simulink model "SimulationOfFurutaL"  (R2017a)
settings: Solver=ode5  StartTime=0.0  StopTime=20  FixedStep=0.0001  RelTol=1e-3  EnableMultiTasking=on
settings Model: Creator=marce  LastModifiedBy=felip
settings DataIOCC: LimitDataPoints=on  SaveFormat=Array
settings OptimizationCC: LifeSpan=inf
settings DebuggingCC: SFUnexpectedBacktrackingDiag=warning  SFNoUnconditionalDefaultTransitionDiag=warning  SFExecutionAtInitializationDiag=none
settings HardwareCC: ProdBitPerPointer=32  ProdBitPerSizeT=32  ProdBitPerPtrDiffT=32  ProdLargestAtomicFloat=None  ProdIntDivRoundTo=Undefined  ProdEndianess=Unspecified  ProdWordSize=32  ProdHWDeviceType=32-bit Generic
settings ModelReferenceCC: PropagateSignalLabelsOutOfModel=off
settings GRTTargetCC: TargetLangStandard=C89/C90 (ANSI)  GeneratePreprocessorConditionals=Disable all
settings ConfigComp: CovMetricSettings=dw  CovHtmlReporting=on  CovSaveCumulativeToWorkspaceVar=on  CovSaveSingleToWorkspaceVar=on  CovExternalEMLEnable=off

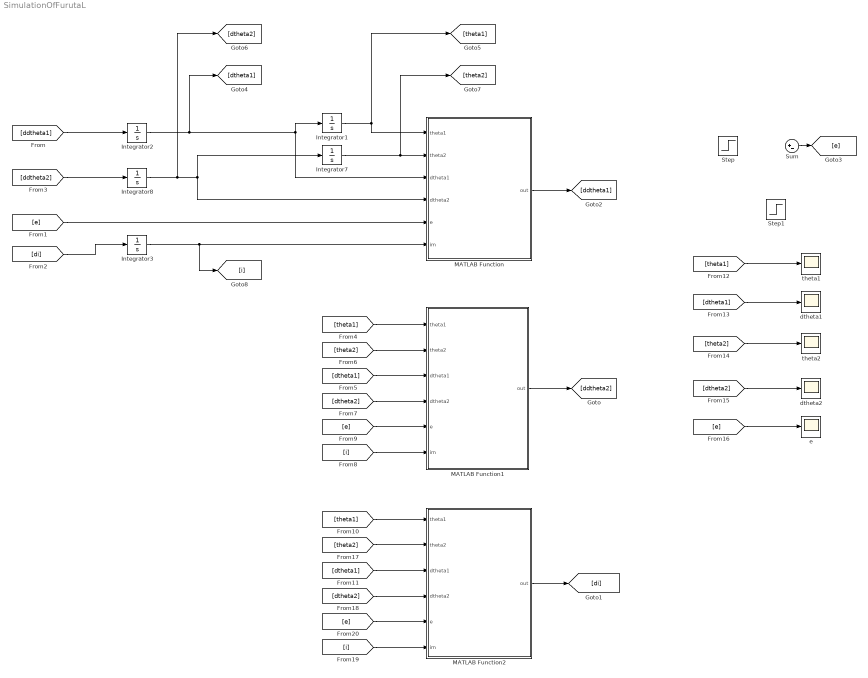
== system SimulationOfFurutaL ==
  Integrator{1..3,8} (4 alike) : Integrator
  Integrator7 : Integrator  InitialCondition=pi*15/180
  MATLAB Function : MATLAB Function  TreatAsAtomicUnit=on
  MATLAB Function1 : MATLAB Function  TreatAsAtomicUnit=on
  MATLAB Function2 : MATLAB Function  TreatAsAtomicUnit=on
  Step : Step  Time=0  After=12  SampleTime=0
  Step1 : Step  Time=1/12  After=12  SampleTime=0
  Sum : Sum  Inputs=|+-
  dtheta1 : Scope
  dtheta2 : Scope
  e : Scope
  theta1 : Scope
  theta2 : Scope
  wires:
  MATLAB Function/1(out) -> [ddtheta1]
  MATLAB Function2/1(out) -> [di]
  MATLAB Function1/1(out) -> [ddtheta2]
  [ddtheta1] -> Integrator2/1
  [ddtheta2] -> Integrator8/1
  Integrator8/1 -> Integrator7/1, MATLAB Function/4(dtheta2), [dtheta2]
  Integrator7/1 -> [theta2], MATLAB Function/2(theta2)
  Sum/1 -> [e]
  Integrator1/1 -> MATLAB Function/1(theta1), [theta1]
  [theta1] -> theta1/1
  [dtheta1] -> dtheta1/1
  [theta2] -> theta2/1
  [dtheta2] -> dtheta2/1
  [e] -> e/1
  Integrator2/1 -> [dtheta1], MATLAB Function/3(dtheta1), Integrator1/1
  [e] -> MATLAB Function/5(e)
  [di] -> Integrator3/1
  Integrator3/1 -> [i], MATLAB Function/6(im)
  [theta1] -> MATLAB Function1/1(theta1)
  [dtheta1] -> MATLAB Function1/3(dtheta1)
  [theta2] -> MATLAB Function1/2(theta2)
  [dtheta2] -> MATLAB Function1/4(dtheta2)
  [i] -> MATLAB Function1/6(im)
  [e] -> MATLAB Function1/5(e)
  [dtheta1] -> MATLAB Function2/3(dtheta1)
  [dtheta2] -> MATLAB Function2/4(dtheta2)
  [theta2] -> MATLAB Function2/2(theta2)
  [theta1] -> MATLAB Function2/1(theta1)
  [e] -> MATLAB Function2/5(e)
  [i] -> MATLAB Function2/6(im)

== matlab function SimulationOfFurutaL/MATLAB Function1 ==
  data: theta1 input; out output; theta2 input; dtheta1 input; dtheta2 input; e input; im input
% function ddtheta2 = fcn(theta1,theta2,dtheta1,dtheta2,e,im)
% coder.extrinsic('solveDdtheta2');
% ddtheta2=0;
% ddtheta2 = solveDdtheta2(theta1,theta2,dtheta1,dtheta2,e,im);

function out=solveDdtheta2(theta1,theta2,dtheta1,dtheta2,e,im)
out =(1431259319741222046139412019291729465658711250000000000000*dtheta2 - 73223699175765104097704098504466175968330259996459663360000*sin(theta2) + 4179825771813674432689680643670944105205968907595153408000*cos(theta2)^2*sin(theta2) + 1328211604542620292753671567216887771948908544000000000000*dtheta1*cos(theta2) - 26855340948310838921835218443053592591014665000000000000000*im*cos(theta2) - 81700523985312009044964891977604498739437398437500000000*dtheta2*cos(theta2)^2 + 67504386807397410253809276909894088519501885448447433849*dtheta1^2*cos(theta2)^3*sin(theta2) - 1182566255742416826397226960059517225138380740493425850080*dtheta1^2*cos(theta2)*sin(theta2) + 148519767147402037084887794151775443283969453160802816400*dtheta2^2*cos(theta2)*sin(theta2) + 200257192730376817043486701661497281910595337930579522120*dtheta1*dtheta2*cos(theta2)^2*sin(theta2))/(2*(108315493778432134648308023899541463893976824135557742312*cos(theta2)^2 - 596598493098508280861020244587343550248245548469369175040))

== matlab function SimulationOfFurutaL/MATLAB Function ==
  data: theta1 input; out output; theta2 input; dtheta1 input; dtheta2 input; e input; im input
% function ddtheta1 = fcn(theta1,theta2,dtheta1,dtheta2,e,im)
% coder.extrinsic('solveDdtheta1');
% ddtheta1=0;
% ddtheta1 = solveDdtheta1(theta1,theta2,dtheta1,dtheta2,e,im);

function out=solveDdtheta1(theta1,theta2,dtheta1,dtheta2,e,im)
out=(225874816564541760468631318756524715309164134400000000000*dtheta1 - 4567002117532915096559827880939460327627204000000000000000*im + 25257176677190688217817535162612333310987843602406424640*dtheta2^2*sin(theta2) - 1549973666070248458619536416033356277909340730299514880000*cos(theta2)*sin(theta2) + 30296396930063072982334500371046219257845273437500000000*dtheta2*cos(theta2) - 25032149091297102130435837707687160238824417241322440265*dtheta1^2*cos(theta2)^2*sin(theta2) + 34055610204731116105864126823653742251992097555156334112*dtheta1*dtheta2*cos(theta2)*sin(theta2))/(2*(27078873444608033662077005974885365973494206033889435578*cos(theta2)^2 - 149149623274627070215255061146835887562061387117342293760))

== matlab function SimulationOfFurutaL/MATLAB Function2 ==
  data: theta1 input; out output; theta2 input; dtheta1 input; dtheta2 input; e input; im input
% function di = fcn(theta1,theta2,dtheta1,dtheta2,e,im)
% coder.extrinsic('solvei');
% di=0;
% di = solvei(theta1,theta2,dtheta1,dtheta2,e,im);

function out= solvei(theta1,theta2,dtheta1,dtheta2,e,im)
out=(4611686018427387904*e)/3782043703712301 - (564129103890148672*dtheta1)/3782043703712301 - (1427316822703276556288*im)/94551092592807525
